simulink model "w2_4"  (R2021a)
settings: Solver=VariableStepAuto  StartTime=0.0  StopTime=10.0  RelTol=1e-3
values from neighbouring files (symbols this model uses):
  b = 3.5077E-6    [data.sldd]    (also in w2_4_1.sldd = 3.5077E-6
  J = 3.2284E-6    [data.sldd]    (also in w2_4_1.sldd = 3.2284E-6
  K = 0.0274    [data.sldd]    (also in w2_4_1.sldd = 0.0274
  L = 2.75E-6    [data.sldd]    (also in w2_4_1.sldd = 2.75E-6
  R = 4.0    [data.sldd]    (also in w2_4_1.sldd = 4.0
settings Model: Creator=AVM  LastModifiedBy=AVM

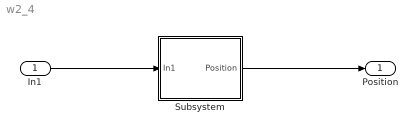
== system w2_4 ==
  In1 : Inport  OutDataTypeStr=double  PortDimensions=1  SampleTime=0
  Subsystem : Subsystem  TreatAsAtomicUnit=on
  Position : Outport
  wires:
  In1/1 -> Subsystem/1(In1)
  Subsystem/1(Position) -> Position/1

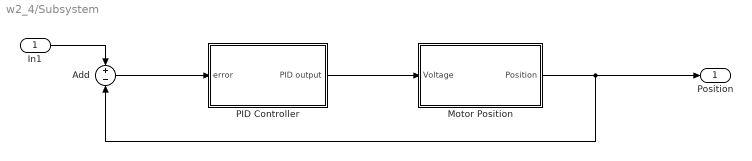
== system w2_4/Subsystem ==
  In1 : Inport  OutDataTypeStr=double  PortDimensions=1  SampleTime=0
  Add : Sum  Inputs=+-
  Motor Position : Subsystem
  PID Controller : Subsystem
  Position : Outport
  wires:
  Add/1 -> PID Controller/1(error)
  Motor Position/1(Position) -> Position/1, Add/2
  PID Controller/1(PID output) -> Motor Position/1(Voltage)
  In1/1 -> Add/1

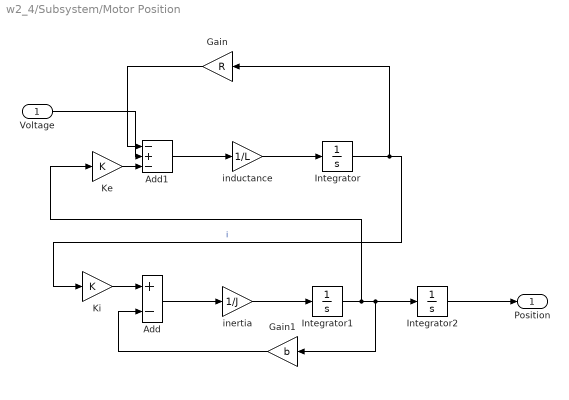
== system w2_4/Subsystem/Motor Position ==
  Voltage : Inport
  Add : Sum  Inputs=+-
  Add1 : Sum  Inputs=-+-
  Gain : Gain  Gain=R
  Gain1 : Gain  Gain=b
  Integrator : Integrator
  Integrator1 : Integrator
  Integrator2 : Integrator
  Ke : Gain  Gain=K
  Ki : Gain  Gain=K
  inductance : Gain  Gain=1/L
  inertia : Gain  Gain=1/J
  Position : Outport
  wires:
  Voltage/1 -> Add1/2
  inertia/1 -> Integrator1/1
  Integrator/1 -> Ki/1, Gain/1  "i"
  inductance/1 -> Integrator/1
  Ke/1 -> Add1/3
  Add1/1 -> inductance/1
  Integrator2/1 -> Position/1
  Ki/1 -> Add/1
  Gain/1 -> Add1/1
  Add/1 -> inertia/1
  Gain1/1 -> Add/2
  Integrator1/1 -> Integrator2/1, Gain1/1, Ke/1

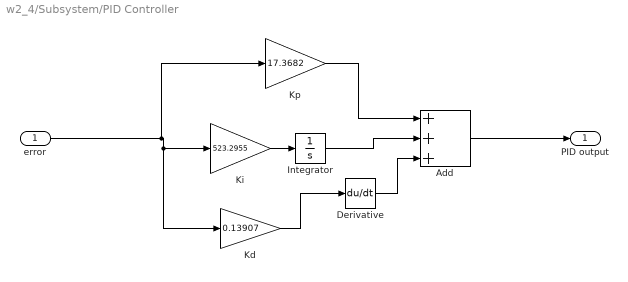
== system w2_4/Subsystem/PID Controller ==
  error : Inport
  Add : Sum  Inputs=+++
  Derivative : Derivative
  Integrator : Integrator
  Kd : Gain  Gain=0.13907
  Ki : Gain  Gain=523.2955
  Kp : Gain  Gain=17.3682
  PID output : Outport
  wires:
  Add/1 -> PID output/1
  error/1 -> Kp/1, Ki/1, Kd/1
  Derivative/1 -> Add/3
  Kd/1 -> Derivative/1
  Kp/1 -> Add/1
  Integrator/1 -> Add/2
  Ki/1 -> Integrator/1
